simulink model "ABS"  (R2022b)
settings: Solver=VariableStepAuto  StartTime=0.0  StopTime=10  RelTol=1e-3
PreLoadFcn:
  | g = 9.81;
  | v0 = 27.77;
  | r_Roue = 0.3;
  | J = 0.5;
  | m = 1000;
  | 
  | Omega_0 = 0;
InitFcn:
  | ABS_config
libraries: slpidlib x3, simulink x2
settings Model: Creator=Youssef ABLALI  LastModifiedBy=Youssef ABLALI

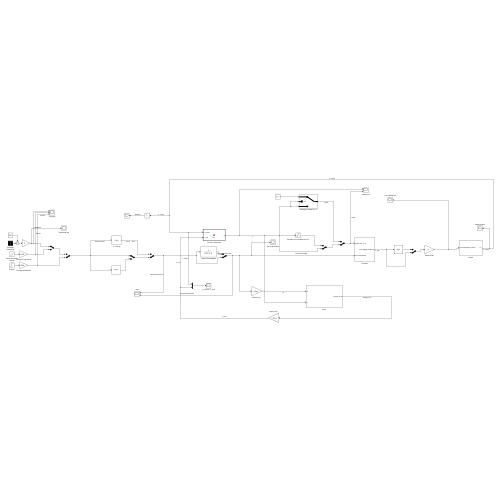
[thumbnail: Simulink's stored preview of the top-level diagram]
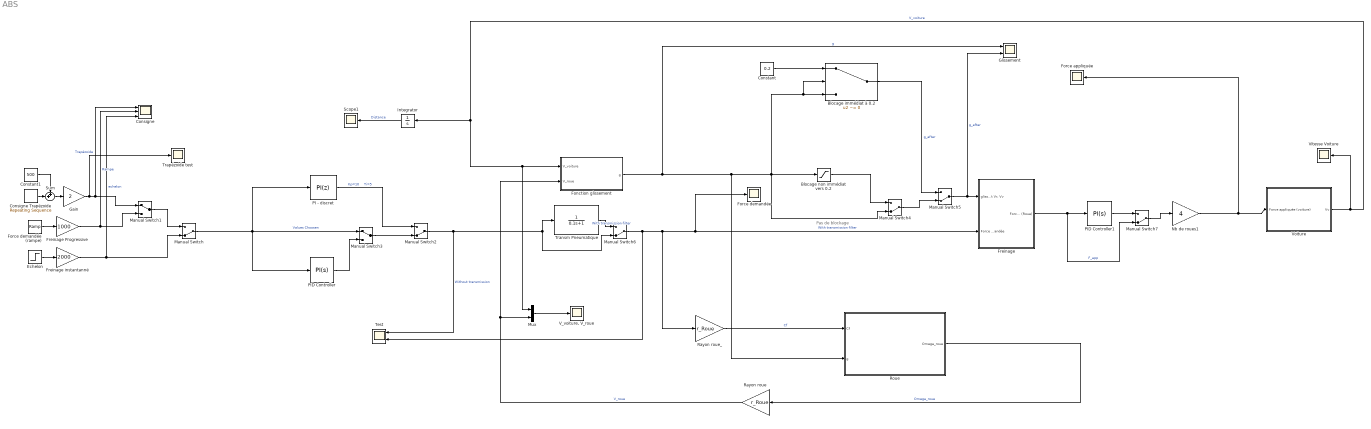
== system ABS ==
  note: Pas de blockage
  Blocage immédiat à 0.2 : Switch  Criteria=u2 ~= 0  SaturateOnIntegerOverflow=off  InputSameDT=off
  Blocage non immédiat vers 0.2 : Saturate
  Consigne : Scope  NumInputPorts=3
  Consigne Trapézoide : simulink/Sources/Repeating Sequence  rep_seq_t=[0 0.1 0.2 0.3 0.4 0.5]  rep_seq_y=[0 1000 1000 1000 0 0]
  Constant : Constant  Value=0.2
  Constant1 : Constant  Value=500
  Echelon : Step  SampleTime=0
  Fonction glissement : MATLAB Function  TreatAsAtomicUnit=on
  Force appliquée : Scope
  Force demandée : Scope
  Force demandée (rampe) : simulink/Sources/Ramp  slope=1  start=0  InitialOutput=0
  Freinage : Subsystem
  Freinage Progressive : Gain  Gain=1000
  Freinage instantanné : Gain  Gain=2000
  Gain : Gain  Gain=2
  Glissement : Scope  NumInputPorts=2
  Integrator : Integrator
  Manual Switch{,2,4..7} (6 alike) : ManualSwitch  CurrentSetting=0
  Manual Switch1 : ManualSwitch
  Manual Switch3 : ManualSwitch
  Mux : Mux  Inputs=2
  Nb de roues1 : Gain  Gain=4
  PI - discret : slpidlib/PID Controller  Controller=PI  Form=Parallel  TimeDomain=Discrete-time  UseExternalTs=off  SampleTime=-1  IntegratorMethod=Forward Euler  FilterMethod=Forward Euler  ControllerParametersSource=internal  P=10  I=5  UseKiTs=off  D=0  N=100  UseFilter=on  TunerSelectOption=Transfer Function Based (PID Tuner App)  InitialConditionSource=internal  InitialConditionForIntegrator=0  InitialConditionForFilter=0  DifferentiatorICPrevScaledInput=0  ExternalReset=none  TrackingMode=off  Kt=1  LimitOutput=off  SatLimitsSource=internal  UpperSaturationLimit=inf  LowerSaturationLimit=-inf  LinearizeAsGain=off  AntiWindupMode=none  Kb=1  LimitIntegrator=off  UpperIntegratorSaturationLimit=inf  LowerIntegratorSaturationLimit=-inf  POutMin=[]  POutMax=[]  IOutMin=[]  IOutMax=[]  DOutMin=[]  DOutMax=[]  NOutMin=[]  NOutMax=[]  SumOutMin=[]  SumOutMax=[]  SaturationOutMin=[]  SaturationOutMax=[]  PParamMin=[]  PParamMax=[]  IParamMin=[]  IParamMax=[]  DParamMin=[]  DParamMax=[]  NParamMin=[]  NParamMax=[]  KbParamMin=[]  KbParamMax=[]  KtParamMin=[]  KtParamMax=[]  KbOutMin=[]  KbOutMax=[]  KtOutMin=[]  KtOutMax=[]  IntegratorOutMin=[]  IntegratorOutMax=[]  FilterOutMin=[]  FilterOutMax=[]  SumI1OutMin=[]  SumI1OutMax=[]  SumI2OutMin=[]  SumI2OutMax=[]  SumI3OutMin=[]  SumI3OutMax=[]  SumI4OutMin=[]  SumI4OutMax=[]  SumDOutMin=[]  SumDOutMax=[]  DifferentiatorOutMin=[]  DifferentiatorOutMax=[]  FilterDiffOutCoefMin=[]  FilterDiffOutCoefMax=[]  ReciprocalOutMin=[]  ReciprocalOutMax=[]  SumDenOutMin=[]  SumDenOutMax=[]  SumNumOutMin=[]  SumNumOutMax=[]  DivideOutMin=[]  DivideOutMax=[]  UdiffTsProdOutMin=[]  UdiffTsProdOutMax=[]  NTsProdOutMin=[]  NTsProdOutMax=[]  UintegralTsProdOutMin=[]  UintegralTsProdOutMax=[]  UngainTsProdOutMin=[]  UngainTsProdOutMax=[]  ClampingZeroOutDataTypeStr=Inherit: Inherit via back propagation  ClampingZeroOutMin=[]  ClampingZeroOutMax=[]  FilterDenConstantOutDataTypeStr=Inherit: Inherit via back propagation  FilterDenConstantOutMin=[]  FilterDenConstantOutMax=[]  PCopyOutDataTypeStr=Inherit: Inherit via back propagation  PCopyOutMin=[]  PCopyOutMax=[]  NCopyOutDataTypeStr=Inherit: Inherit via back propagation  NCopyOutMin=[]  NCopyOutMax=[]  IntegratorContinuousStateAttributes=''  IntegratorStateMustResolveToSignalObject=off  IntegratorRTWStateStorageClass=Auto  FilterContinuousStateAttributes=''  FilterStateMustResolveToSignalObject=off  FilterRTWStateStorageClass=Auto  ParallelPVariant=InternalParameters  IdealPVariant=Disabled  IVariant=InternalParameters  DVariant=Disabled  IntegratorVariant=Discrete  SatVariant=Disabled  AWVariant=Passthrough  PCopyVariant=Disabled  TRVariant=Disabled  FdbkBlocksVariant=Forward  IdealPFdbkVariant=Disabled  SatFdbkVariant=Disabled  DerivativeFilterVariant=Disabled  NVariant=Disabled  NCopyVariant=Disabled_SignalSpec  FilterICVariant=Disabled  IntegratorICVariant=InternalICs  ExternalResetVariant=Disabled  TRSumVariant=Passthrough  SumFdbkVariant=Disabled  SumVariant=Sum_PI  TsampFilterVariant=InternalTs  TsampNgainVariant=Passthrough  TsampIntegralVariant=Passthrough  ExternalSaturationOutDataTypeStr=Inherit: Same as second input
      settings: LibrarySourceBlock=simulink/Discrete/Discrete PID Controller
  PID Controller : slpidlib/PID Controller  Controller=PI  Form=Parallel  TimeDomain=Continuous-time  UseExternalTs=off  SampleTime=-1  IntegratorMethod=Forward Euler  FilterMethod=Forward Euler  ControllerParametersSource=internal  P=10  I=0.1  UseKiTs=off  D=3  N=100  UseFilter=on  TunerSelectOption=Transfer Function Based (PID Tuner App)  InitialConditionSource=internal  InitialConditionForIntegrator=0  InitialConditionForFilter=0  DifferentiatorICPrevScaledInput=0  ExternalReset=none  TrackingMode=off  Kt=1  LimitOutput=off  SatLimitsSource=internal  UpperSaturationLimit=inf  LowerSaturationLimit=-inf  LinearizeAsGain=on  AntiWindupMode=none  Kb=1  LimitIntegrator=off  UpperIntegratorSaturationLimit=inf  LowerIntegratorSaturationLimit=-inf  POutMin=[]  POutMax=[]  IOutMin=[]  IOutMax=[]  DOutMin=[]  DOutMax=[]  NOutMin=[]  NOutMax=[]  SumOutMin=[]  SumOutMax=[]  SaturationOutMin=[]  SaturationOutMax=[]  PParamMin=[]  PParamMax=[]  IParamMin=[]  IParamMax=[]  DParamMin=[]  DParamMax=[]  NParamMin=[]  NParamMax=[]  KbParamMin=[]  KbParamMax=[]  KtParamMin=[]  KtParamMax=[]  KbOutMin=[]  KbOutMax=[]  KtOutMin=[]  KtOutMax=[]  IntegratorOutMin=[]  IntegratorOutMax=[]  FilterOutMin=[]  FilterOutMax=[]  SumI1OutMin=[]  SumI1OutMax=[]  SumI2OutMin=[]  SumI2OutMax=[]  SumI3OutMin=[]  SumI3OutMax=[]  SumI4OutMin=[]  SumI4OutMax=[]  SumDOutMin=[]  SumDOutMax=[]  DifferentiatorOutMin=[]  DifferentiatorOutMax=[]  FilterDiffOutCoefMin=[]  FilterDiffOutCoefMax=[]  ReciprocalOutMin=[]  ReciprocalOutMax=[]  SumDenOutMin=[]  SumDenOutMax=[]  SumNumOutMin=[]  SumNumOutMax=[]  DivideOutMin=[]  DivideOutMax=[]  UdiffTsProdOutMin=[]  UdiffTsProdOutMax=[]  NTsProdOutMin=[]  NTsProdOutMax=[]  UintegralTsProdOutMin=[]  UintegralTsProdOutMax=[]  UngainTsProdOutMin=[]  UngainTsProdOutMax=[]  ClampingZeroOutDataTypeStr=Inherit: Inherit via back propagation  ClampingZeroOutMin=[]  ClampingZeroOutMax=[]  FilterDenConstantOutDataTypeStr=Inherit: Inherit via back propagation  FilterDenConstantOutMin=[]  FilterDenConstantOutMax=[]  PCopyOutDataTypeStr=Inherit: Inherit via back propagation  PCopyOutMin=[]  PCopyOutMax=[]  NCopyOutDataTypeStr=Inherit: Inherit via back propagation  NCopyOutMin=[]  NCopyOutMax=[]  IntegratorContinuousStateAttributes=''  IntegratorStateMustResolveToSignalObject=off  IntegratorRTWStateStorageClass=Auto  FilterContinuousStateAttributes=''  FilterStateMustResolveToSignalObject=off  FilterRTWStateStorageClass=Auto  ParallelPVariant=InternalParameters  IdealPVariant=Disabled  IVariant=InternalParameters  DVariant=Disabled  IntegratorVariant=Continuous  SatVariant=Disabled  AWVariant=Passthrough  PCopyVariant=Disabled  TRVariant=Disabled  FdbkBlocksVariant=Forward  IdealPFdbkVariant=Disabled  SatFdbkVariant=Disabled  DerivativeFilterVariant=Disabled  NVariant=Disabled  NCopyVariant=Disabled_SignalSpec  FilterICVariant=Disabled  IntegratorICVariant=InternalICs  ExternalResetVariant=Disabled  TRSumVariant=Passthrough  SumFdbkVariant=Disabled  SumVariant=Sum_PI  TsampFilterVariant=InternalTs  TsampNgainVariant=Passthrough  TsampIntegralVariant=Passthrough  ExternalSaturationOutDataTypeStr=Inherit: Same as second input
  PID Controller1 : slpidlib/PID Controller  Controller=PI  Form=Parallel  TimeDomain=Continuous-time  UseExternalTs=off  SampleTime=-1  IntegratorMethod=Forward Euler  FilterMethod=Forward Euler  ControllerParametersSource=internal  P=10  I=0.1  UseKiTs=off  D=3  N=100  UseFilter=on  TunerSelectOption=Transfer Function Based (PID Tuner App)  InitialConditionSource=internal  InitialConditionForIntegrator=0  InitialConditionForFilter=0  DifferentiatorICPrevScaledInput=0  ExternalReset=none  TrackingMode=off  Kt=1  LimitOutput=off  SatLimitsSource=internal  UpperSaturationLimit=inf  LowerSaturationLimit=-inf  LinearizeAsGain=on  AntiWindupMode=none  Kb=1  LimitIntegrator=off  UpperIntegratorSaturationLimit=inf  LowerIntegratorSaturationLimit=-inf  POutMin=[]  POutMax=[]  IOutMin=[]  IOutMax=[]  DOutMin=[]  DOutMax=[]  NOutMin=[]  NOutMax=[]  SumOutMin=[]  SumOutMax=[]  SaturationOutMin=[]  SaturationOutMax=[]  PParamMin=[]  PParamMax=[]  IParamMin=[]  IParamMax=[]  DParamMin=[]  DParamMax=[]  NParamMin=[]  NParamMax=[]  KbParamMin=[]  KbParamMax=[]  KtParamMin=[]  KtParamMax=[]  KbOutMin=[]  KbOutMax=[]  KtOutMin=[]  KtOutMax=[]  IntegratorOutMin=[]  IntegratorOutMax=[]  FilterOutMin=[]  FilterOutMax=[]  SumI1OutMin=[]  SumI1OutMax=[]  SumI2OutMin=[]  SumI2OutMax=[]  SumI3OutMin=[]  SumI3OutMax=[]  SumI4OutMin=[]  SumI4OutMax=[]  SumDOutMin=[]  SumDOutMax=[]  DifferentiatorOutMin=[]  DifferentiatorOutMax=[]  FilterDiffOutCoefMin=[]  FilterDiffOutCoefMax=[]  ReciprocalOutMin=[]  ReciprocalOutMax=[]  SumDenOutMin=[]  SumDenOutMax=[]  SumNumOutMin=[]  SumNumOutMax=[]  DivideOutMin=[]  DivideOutMax=[]  UdiffTsProdOutMin=[]  UdiffTsProdOutMax=[]  NTsProdOutMin=[]  NTsProdOutMax=[]  UintegralTsProdOutMin=[]  UintegralTsProdOutMax=[]  UngainTsProdOutMin=[]  UngainTsProdOutMax=[]  ClampingZeroOutDataTypeStr=Inherit: Inherit via back propagation  ClampingZeroOutMin=[]  ClampingZeroOutMax=[]  FilterDenConstantOutDataTypeStr=Inherit: Inherit via back propagation  FilterDenConstantOutMin=[]  FilterDenConstantOutMax=[]  PCopyOutDataTypeStr=Inherit: Inherit via back propagation  PCopyOutMin=[]  PCopyOutMax=[]  NCopyOutDataTypeStr=Inherit: Inherit via back propagation  NCopyOutMin=[]  NCopyOutMax=[]  IntegratorContinuousStateAttributes=''  IntegratorStateMustResolveToSignalObject=off  IntegratorRTWStateStorageClass=Auto  FilterContinuousStateAttributes=''  FilterStateMustResolveToSignalObject=off  FilterRTWStateStorageClass=Auto  ParallelPVariant=InternalParameters  IdealPVariant=Disabled  IVariant=InternalParameters  DVariant=Disabled  IntegratorVariant=Continuous  SatVariant=Disabled  AWVariant=Passthrough  PCopyVariant=Disabled  TRVariant=Disabled  FdbkBlocksVariant=Forward  IdealPFdbkVariant=Disabled  SatFdbkVariant=Disabled  DerivativeFilterVariant=Disabled  NVariant=Disabled  NCopyVariant=Disabled_SignalSpec  FilterICVariant=Disabled  IntegratorICVariant=InternalICs  ExternalResetVariant=Disabled  TRSumVariant=Passthrough  SumFdbkVariant=Disabled  SumVariant=Sum_PI  TsampFilterVariant=InternalTs  TsampNgainVariant=Passthrough  TsampIntegralVariant=Passthrough  ExternalSaturationOutDataTypeStr=Inherit: Same as second input
  Rayon roue : Gain  Gain=r_Roue
  Rayon roue_ : Gain  Gain=r_Roue
  Roue : Subsystem
  Scope1 : Scope
  Sum : Sum  Inputs=++|
  Test : Scope  NumInputPorts=2
  Transm Pneumatique : TransferFcn  Denominator=[0.1 1]
  Trapézoide test : Scope
  "V_voiture, V_roue" : Scope
  Vitesse Voiture : Scope
  Voiture : Subsystem
  wires:
  Voiture/1("Vv ") -> Integrator/1, Mux/1, Fonction glissement/1(V_voiture), Vitesse Voiture/1  "V_voiture"
  Rayon roue_/1 -> Roue/1(Cf)  "Cf"
  Fonction glissement/1(g) -> Glissement/1, Blocage immédiat à 0.2/2, Blocage immédiat à 0.2/3, Blocage non immédiat vers 0.2/1, Manual Switch4/2, Roue/2(g)  "g"
  Roue/1(Omega_roue) -> Rayon roue/1  "Omega_roue"
  Manual Switch1/1 -> Manual Switch/1
  Echelon/1 -> Freinage instantanné/1
  Force demandée (rampe)/1 -> Freinage Progressive/1
  Rayon roue/1 -> Fonction glissement/2(V_roue), Mux/2  "V_roue"
  Gain/1 -> Trapézoide test/1, Consigne/1, Manual Switch1/1  "Trapézoide"
  Freinage Progressive/1 -> Consigne/2, Manual Switch1/2  "Rampe"
  Freinage instantanné/1 -> Manual Switch/2, Consigne/3  "echelon"
  Mux/1 -> "V_voiture, V_roue"/1
  Manual Switch6/1 -> Test/2, Freinage/2(Force demandée), Force demandée/1, Rayon roue_/1  "With transmission filter"
  Manual Switch/1 -> PID Controller/1, PI - discret/1, Manual Switch3/1  "Values Choosen"
  Manual Switch2/1 -> Manual Switch6/2, Transm Pneumatique/1, Test/1  "Without transmission"
  Manual Switch3/1 -> Manual Switch2/2
  PID Controller/1 -> Manual Switch3/2
  PI - discret/1 -> Manual Switch2/1  "Kp=10     Ti=5"
  Integrator/1 -> Scope1/1  "Distance"
  Blocage immédiat à 0.2/1 -> Manual Switch5/1  "g_after"
  Constant/1 -> Blocage immédiat à 0.2/1
  Manual Switch5/1 -> Glissement/2, Freinage/1("glissement Vr, Vv")  "g_after"
  Blocage non immédiat vers 0.2/1 -> Manual Switch4/1
  Manual Switch4/1 -> Manual Switch5/2
  Transm Pneumatique/1 -> Manual Switch6/1  "With transmission filter"
  Sum/1 -> Gain/1
  Consigne Trapézoide/1 -> Sum/2
  Constant1/1 -> Sum/1
  Nb de roues1/1 -> Force appliquée/1, Voiture/1(Force appliquée (voiture))
  Manual Switch7/1 -> Nb de roues1/1
  PID Controller1/1 -> Manual Switch7/1
  Freinage/1(Force Appliquée (Roue)) -> Manual Switch7/2, PID Controller1/1  "F_app"

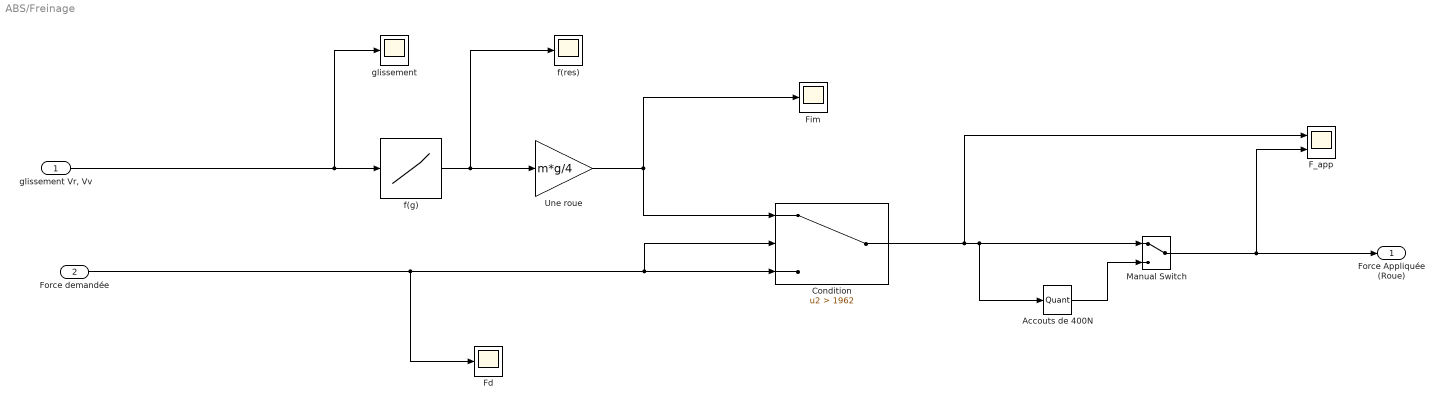
== system ABS/Freinage ==
  "glissement Vr, Vv" : Inport
  Force demandée : Inport  Port=2
  Accouts de 400N : Quantizer  QuantizationInterval=400
  "Condition " : Switch  Criteria=u2 > Threshold  Threshold=1962  SaturateOnIntegerOverflow=off  InputSameDT=off
  F_app : Scope  NumInputPorts=2
  Fd : Scope
  Fim : Scope
  Manual Switch : ManualSwitch
  Une roue : Gain  Gain=m*g/4
  f(g) : Lookup_n-D  NumberOfTableDimensions=1  BreakpointsForDimension1=[0,0.1,0.2,0.3,0.4,0.5,0.6,0.7,0.8,0.9,1.0]  Table=[0.0,0.85,0.95,0.78,0.73,0.7,0.68,0.66,0.64,0.62,0.61]  InternalRulePriority=Speed  RndMeth=Simplest
  f(res) : Scope
  glissement : Scope
  Force Appliquée (Roue) : Outport  VectorParamsAs1DForOutWhenUnconnected=off
  wires:
  f(g)/1 -> f(res)/1, Une roue/1
  Une roue/1 -> "Condition "/1, Fim/1
  Force demandée/1 -> Fd/1, "Condition "/3, "Condition "/2
  "glissement Vr, Vv"/1 -> glissement/1, f(g)/1
  Manual Switch/1 -> F_app/2, Force Appliquée (Roue)/1
  "Condition "/1 -> F_app/1, Accouts de 400N/1, Manual Switch/1
  Accouts de 400N/1 -> Manual Switch/2

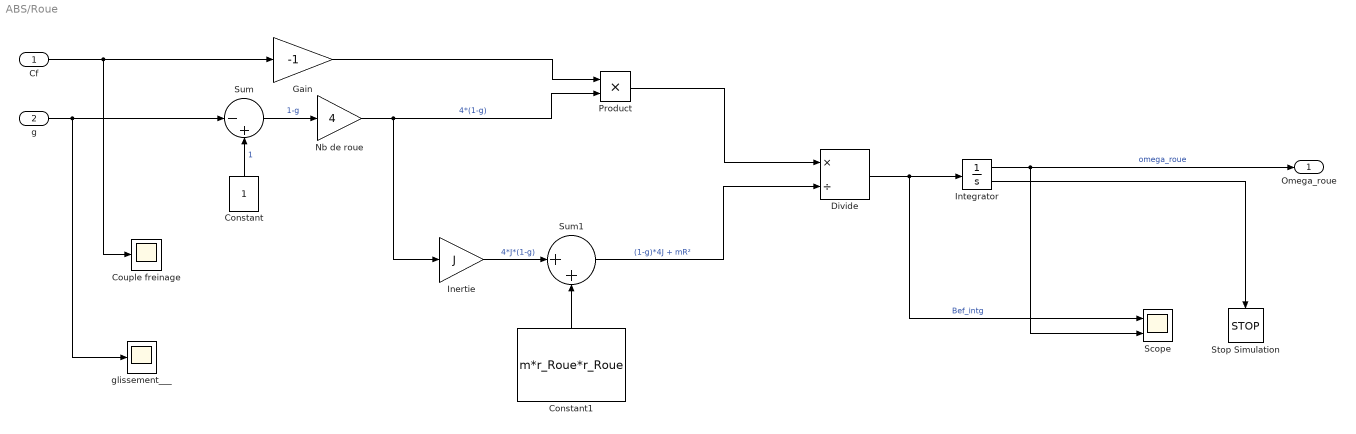
== system ABS/Roue ==
  Cf : Inport
  g : Inport  Port=2
  Constant : Constant
  Constant1 : Constant  Value=m*r_Roue*r_Roue
  Couple freinage : Scope
  Divide : Product  Inputs=*/
  Gain : Gain  Gain=-1
  Inertie : Gain  Gain=J
  Integrator : Integrator  InitialCondition=Omega_0  LimitOutput=on  LowerSaturationLimit=0  ShowSaturationPort=on
  Nb de roue : Gain  Gain=4
  Product : Product
  Scope : Scope  NumInputPorts=2
  Stop Simulation : Stop
  Sum : Sum  Inputs=|-+
  Sum1 : Sum  Inputs=|++
  glissement___ : Scope
  Omega_roue : Outport
  wires:
  Inertie/1 -> Sum1/1  "4*J*(1-g)"
  Sum/1 -> Nb de roue/1  "1-g"
  Sum1/1 -> Divide/2  "(1-g)*4J + mR²"
  Constant1/1 -> Sum1/2
  Product/1 -> Divide/1
  Constant/1 -> Sum/2  "1"
  Divide/1 -> Scope/1, Integrator/1  "Bef_intg"
  Nb de roue/1 -> Inertie/1, Product/2  "4*(1-g)"
  g/1 -> glissement___/1, Sum/1
  Cf/1 -> Couple freinage/1, Gain/1
  Integrator/1 -> Scope/2, Omega_roue/1  "omega_roue"
  Gain/1 -> Product/1
  Integrator/2 -> Stop Simulation/1

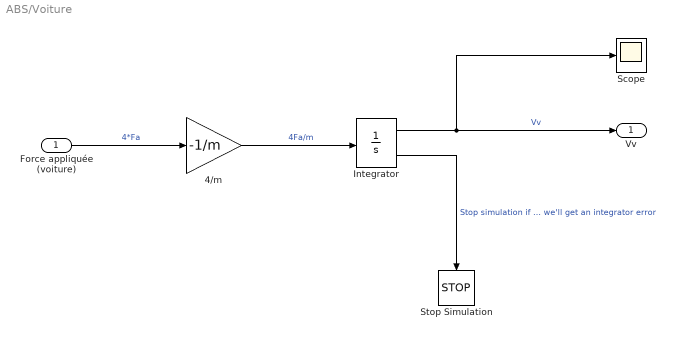
== system ABS/Voiture ==
  Force appliquée (voiture) : Inport
  4/m : Gain  Gain=-1/m
  Integrator : Integrator  InitialCondition=v0  LimitOutput=on  LowerSaturationLimit=0  ShowSaturationPort=on
  Scope : Scope
  Stop Simulation : Stop
  "Vv " : Outport
  wires:
  Force appliquée (voiture)/1 -> 4/m/1  "4*Fa"
  4/m/1 -> Integrator/1  "4Fa/m"
  Integrator/1 -> Scope/1, "Vv "/1  "Vv"
  Integrator/2 -> Stop Simulation/1  "Stop simulation if 0 is reached otherwise, we'll get an integrator error"

== matlab function ABS/Fonction glissement ==
  data: V_voiture input; V_roue input; g output
function g = fcn(V_voiture,V_roue)

g = (V_voiture - V_roue)/V_voiture;
